simulink model "bicycle_sim"  (Simulink 10.2)
settings: Solver=VariableStepAuto  StartTime=0.0  StopTime=30  RelTol=1e-3
values from neighbouring files (symbols this model uses):
  a = 4    [bicycle.m]    (also in matlab.mat)
  d = 0.01    [bicycle.m]    (also in matlab.mat)
  Kp = 0.4    [bicycle.m]    (also in matlab.mat)
  Kth = 1.1    [bicycle.m]    (also in matlab.mat)
  Kx = 15    [bicycle.m]    (also in matlab.mat)
  Ky = 15    [bicycle.m]    (also in matlab.mat)
  L = 0.5    [bicycle.m]    (also in matlab.mat)
  theta0 = pi/2    (= 1.57079632679)    [bicycle.m]    (also in matlab.mat)
  w = 0.1    [bicycle.m]    (also in matlab.mat)
  x0 = a    (= 4)    [bicycle.m]    (also in matlab.mat)
  y0 = 0    [bicycle.m]    (also in matlab.mat)
libraries: simulink_extras x2
settings Model: Creator=olivier  LastModifiedBy=yukisaito
settings SolverCC: ZeroCrossAlgorithm=Adaptive
settings DataIOCC: SaveFormat=Dataset  SignalLoggingSaveFormat=Dataset
settings OptimizationCC: LifeSpan=auto
settings DebuggingCC: UnderspecifiedInitializationDetection=Simplified  MergeDetectMultiDrivingBlocksExec=error  MaskedZcDiagnostic=none  FcnCallInpInsideContextMsg=error  SFUnexpectedBacktrackingDiag=error  SFNoUnconditionalDefaultTransitionDiag=error  SFExecutionAtInitializationDiag=warning
settings HardwareCC: ProdBitPerPointer=64  ProdBitPerSizeT=64  ProdBitPerPtrDiffT=64  ProdLargestAtomicFloat=Float  ProdIntDivRoundTo=Zero  ProdEndianess=LittleEndian  ProdWordSize=64  ProdHWDeviceType=Intel->x86-64 (Windows64)
settings ModelReferenceCC: PropagateSignalLabelsOutOfModel=on
settings SFSimCC: SimUseLocalCustomCode=on
settings RTWCC: RTWUseLocalCustomCode=on
settings CodeAppCC: StateflowObjectComments=off
settings GRTTargetCC: TargetLangStandard=C99 (ISO)  CombineOutputUpdateFcns=on  GRTInterface=off
settings ConfigComp: CovMetricSettings=dwe  CovSaveCumulativeToWorkspaceVar=off  CovSaveSingleToWorkspaceVar=off  CovExternalEMLEnable=on

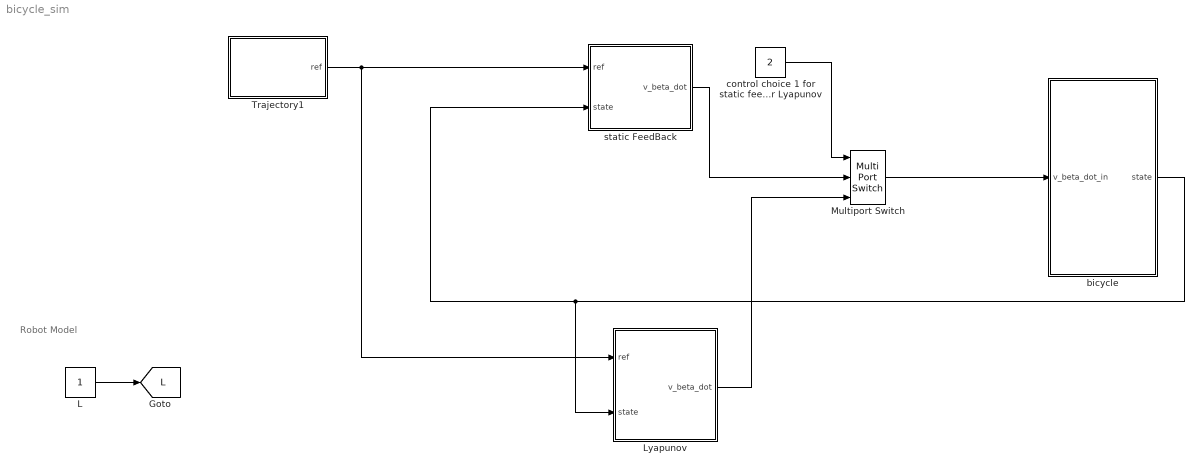
== system bicycle_sim ==
  note: Robot Model
  L : Constant
  Lyapunov : Subsystem
  Multiport Switch : MultiPortSwitch  Inputs=2
  Trajectory1 : Subsystem  TreatAsAtomicUnit=on
  bicycle : Subsystem  mask{L_error=0, radius_error=0, omega_max=100, beta_max=45, beta_dot_max=50}
      mask prompts: L_error "L error in percent"; radius_error "Radius error in percent"; omega_max "Max Rotation Velocity"; beta_max "Max Orientation"; beta_dot_max "Max Orientation Velocity"
  control choice 1 for static feedback 2 for Lyapunov : Constant  Value=2
  static FeedBack : Subsystem
  tag scope: L=global
  wires:
  Lyapunov/1(v_beta_dot) -> Multiport Switch/3
  static FeedBack/1(v_beta_dot) -> Multiport Switch/2
  L/1 -> [L]
  Trajectory1/1(ref) -> Lyapunov/1(ref), static FeedBack/1(ref)
  bicycle/1(state) -> Lyapunov/2(state), static FeedBack/2(state)
  control choice 1 for static feedback 2 for Lyapunov/1 -> Multiport Switch/1
  Multiport Switch/1 -> bicycle/1(v_beta_dot_in)

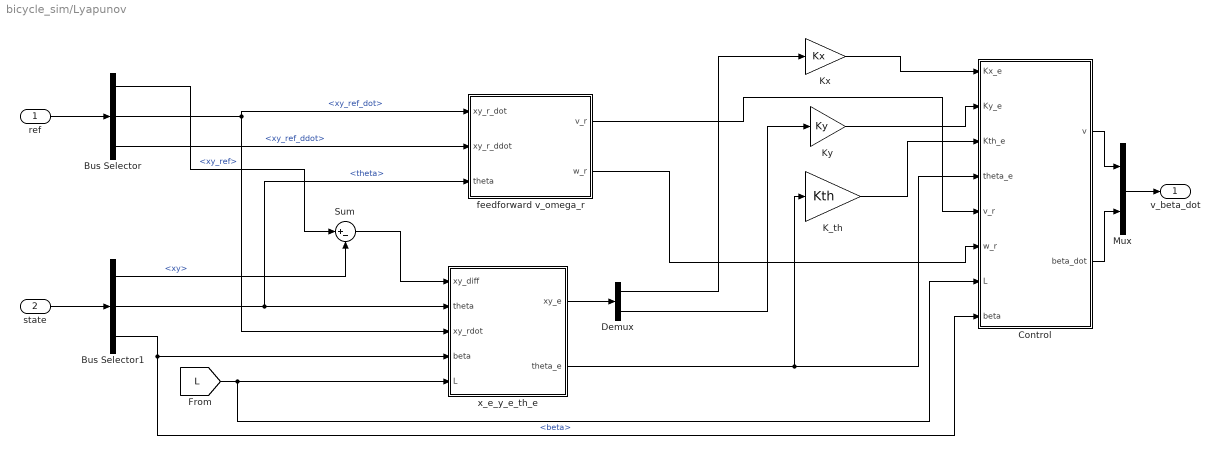
== system bicycle_sim/Lyapunov ==
  ref : Inport
  state : Inport  Port=2
  Bus Selector : BusSelector  OutputSignals=xy_ref,xy_ref_dot,xy_ref_ddot
  Bus Selector1 : BusSelector  OutputSignals=xy,theta,beta
  Control : MATLAB Function  TreatAsAtomicUnit=on
  Demux : Demux  Outputs=2
  K_th : Gain  Gain=Kth
  Kx : Gain  Gain=Kx
  Ky : Gain  Gain=Ky
  Mux : Mux  Inputs=2
  Sum : Sum  Inputs=|+-
  feedforward v_omega_r : MATLAB Function  TreatAsAtomicUnit=on
  x_e_y_e_th_e : MATLAB Function  TreatAsAtomicUnit=on
  v_beta_dot : Outport
  wires:
  state/1 -> Bus Selector1/1
  Demux/1 -> Kx/1
  Bus Selector/2 -> x_e_y_e_th_e/3(xy_rdot), feedforward v_omega_r/1(xy_r_dot)  "<xy_ref_dot>"
  Ky/1 -> Control/2(Ky_e)
  ref/1 -> Bus Selector/1
  Bus Selector/1 -> Sum/1  "<xy_ref>"
  Mux/1 -> v_beta_dot/1
  K_th/1 -> Control/3(Kth_e)
  [L] -> Control/7(L), x_e_y_e_th_e/5(L)
  Demux/2 -> Ky/1
  feedforward v_omega_r/2(w_r) -> Control/6(w_r)
  Sum/1 -> x_e_y_e_th_e/1(xy_diff)
  x_e_y_e_th_e/2(theta_e) -> Control/4(theta_e), K_th/1
  Kx/1 -> Control/1(Kx_e)
  Bus Selector1/1 -> Sum/2  "<xy>"
  Control/1(v) -> Mux/1
  Bus Selector1/2 -> feedforward v_omega_r/3(theta), x_e_y_e_th_e/2(theta)  "<theta>"
  x_e_y_e_th_e/1(xy_e) -> Demux/1
  feedforward v_omega_r/1(v_r) -> Control/5(v_r)
  Bus Selector1/3 -> Control/8(beta), x_e_y_e_th_e/4(beta)  "<beta>"
  Bus Selector/3 -> feedforward v_omega_r/2(xy_r_ddot)  "<xy_ref_ddot>"
  Control/2(beta_dot) -> Mux/2

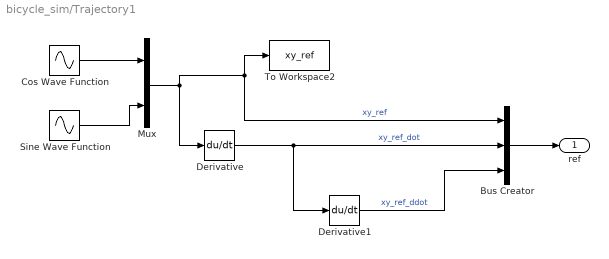
== system bicycle_sim/Trajectory1 ==
  Bus Creator : BusCreator  Inputs=3
  Cos Wave Function : Sin  Amplitude=a  Frequency=w  Phase=pi/2  SampleTime=0
  Derivative : Derivative
  Derivative1 : Derivative
  Mux : Mux  Inputs=2
  Sine Wave Function : Sin  Amplitude=a  Frequency=w  SampleTime=0
  To Workspace2 : ToWorkspace  VariableName=xy_ref  SampleTime=-1
      settings: Save2DSignal=2-D array (concatenate along first dimension)
  ref : Outport  VectorParamsAs1DForOutWhenUnconnected=off
  wires:
  Bus Creator/1 -> ref/1
  Mux/1 -> Derivative/1, Bus Creator/1, To Workspace2/1  "xy_ref"
  Derivative/1 -> Bus Creator/2, Derivative1/1  "xy_ref_dot"
  Derivative1/1 -> Bus Creator/3  "xy_ref_ddot"
  Sine Wave Function/1 -> Mux/2
  Cos Wave Function/1 -> Mux/1

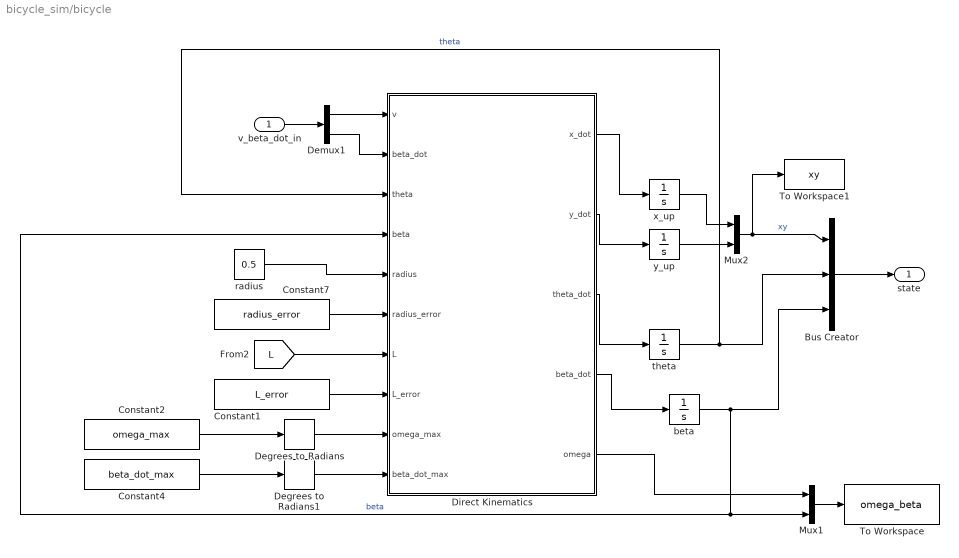
== system bicycle_sim/bicycle ==
  v_beta_dot_in : Inport
  Bus Creator : BusCreator  Inputs=3
  Constant1 : Constant  Value=L_error
  Constant2 : Constant  Value=omega_max
  Constant4 : Constant  Value=beta_dot_max
  Constant7 : Constant  Value=radius_error
  Degrees to Radians : simulink_extras/Transformations/Degrees to Radians
  Degrees to Radians1 : simulink_extras/Transformations/Degrees to Radians
  Demux1 : Demux  Outputs=2
  Direct Kinematics : MATLAB Function  TreatAsAtomicUnit=on
  Mux1 : Mux  Inputs=2
  Mux2 : Mux  Inputs=2
  To Workspace : ToWorkspace  VariableName=omega_beta  SampleTime=-1
      settings: Save2DSignal=2-D array (concatenate along first dimension)
  To Workspace1 : ToWorkspace  VariableName=xy  SampleTime=-1
      settings: Save2DSignal=2-D array (concatenate along first dimension)
  beta : Integrator  LimitOutput=on  UpperSaturationLimit=beta_max*pi/180  LowerSaturationLimit=-beta_max*pi/180
  radius : Constant  Value=0.5
  theta : Integrator  InitialCondition=theta0
  x_up : Integrator  InitialCondition=x0
  y_up : Integrator  InitialCondition=y0
  state : Outport  VectorParamsAs1DForOutWhenUnconnected=off
  wires:
  Direct Kinematics/2(y_dot) -> y_up/1
  Direct Kinematics/1(x_dot) -> x_up/1
  x_up/1 -> Mux2/1
  y_up/1 -> Mux2/2
  Mux2/1 -> Bus Creator/1, To Workspace1/1  "xy"
  Bus Creator/1 -> state/1
  v_beta_dot_in/1 -> Demux1/1
  Demux1/1 -> Direct Kinematics/1(v)
  [L] -> Direct Kinematics/7(L)
  Constant1/1 -> Direct Kinematics/8(L_error)
  Constant7/1 -> Direct Kinematics/6(radius_error)
  Direct Kinematics/3(theta_dot) -> theta/1
  Direct Kinematics/4(beta_dot) -> beta/1
  theta/1 -> Direct Kinematics/3(theta), Bus Creator/2  "theta"
  beta/1 -> Direct Kinematics/4(beta), Mux1/2, Bus Creator/3  "beta"
  Constant2/1 -> Degrees to Radians/1
  Constant4/1 -> Degrees to Radians1/1
  Direct Kinematics/5(omega) -> Mux1/1
  Mux1/1 -> To Workspace/1
  radius/1 -> Direct Kinematics/5(radius)
  Demux1/2 -> Direct Kinematics/2("beta_dot ")
  Degrees to Radians/1 -> Direct Kinematics/9(omega_max)
  Degrees to Radians1/1 -> Direct Kinematics/10(beta_dot_max)

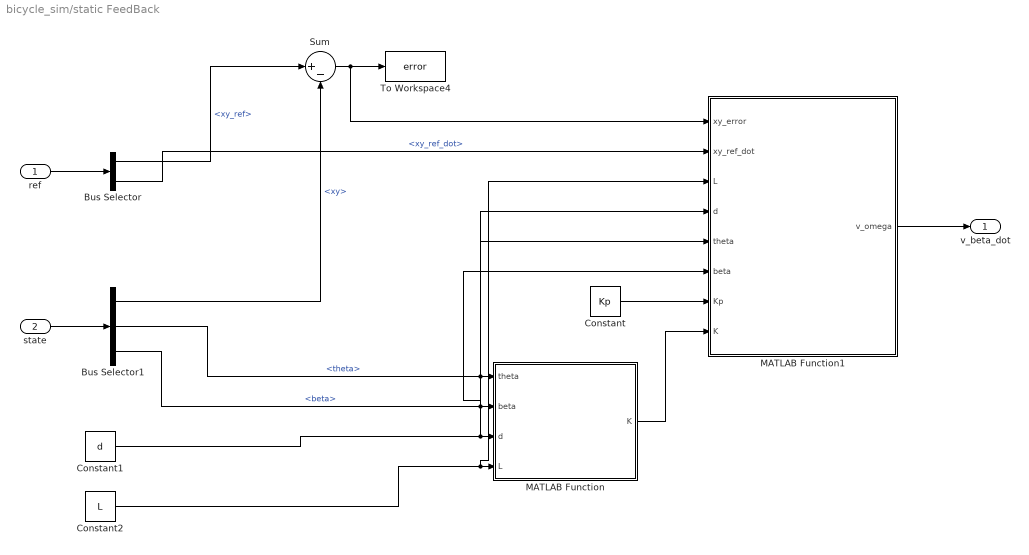
== system bicycle_sim/static FeedBack ==
  ref : Inport
  state : Inport  Port=2
  Bus Selector : BusSelector  OutputSignals=xy_ref,xy_ref_dot
  Bus Selector1 : BusSelector  OutputSignals=xy,theta,beta
  Constant : Constant  Value=Kp
  Constant1 : Constant  Value=d
  Constant2 : Constant  Value=L
  MATLAB Function : MATLAB Function  TreatAsAtomicUnit=on
  MATLAB Function1 : MATLAB Function  TreatAsAtomicUnit=on
  Sum : Sum  Inputs=|+-
  To Workspace4 : ToWorkspace  VariableName=error  SampleTime=-1
      settings: Save2DSignal=2-D array (concatenate along first dimension)
  v_beta_dot : Outport  VectorParamsAs1DForOutWhenUnconnected=off
  wires:
  Sum/1 -> MATLAB Function1/1(xy_error), To Workspace4/1
  ref/1 -> Bus Selector/1
  state/1 -> Bus Selector1/1
  Bus Selector/1 -> Sum/1  "<xy_ref>"
  Bus Selector1/3 -> MATLAB Function1/6(beta), MATLAB Function/2(beta)  "<beta>"
  Bus Selector1/2 -> MATLAB Function1/5(theta), MATLAB Function/1(theta)  "<theta>"
  Bus Selector1/1 -> Sum/2  "<xy>"
  Bus Selector/2 -> MATLAB Function1/2(xy_ref_dot)  "<xy_ref_dot>"
  Constant1/1 -> MATLAB Function1/4(d), MATLAB Function/3(d)
  Constant2/1 -> MATLAB Function1/3(L), MATLAB Function/4(L)
  MATLAB Function/1(K) -> MATLAB Function1/8(K)
  MATLAB Function1/1(v_omega) -> v_beta_dot/1
  Constant/1 -> MATLAB Function1/7(Kp)

== matlab function bicycle/Direct Kinematics ==
  data: v input double; beta_dot input double; x_dot output double; theta input double; beta input double; radius input double; radius_error input double; L input double; L_error input double; omega_max input double; beta_dot_max input double; y_dot output double; theta_dot output double; beta_dot output double; omega output double
function [x_dot, y_dot, theta_dot, beta_dot, omega]  = dk(v, beta_dot, theta, beta, radius, radius_error, L, L_error, omega_max, beta_dot_max)

% commanded wheel rotation velocity
omega = v/radius;
omega = max(-omega_max, min(omega, omega_max));

% actual linear velocity
v = (1+radius_error*0.01)*radius * omega;

% actual L value
L = (1+L_error*0.01)*L;

x_dot = v*cos(theta)*cos(beta);
y_dot = v*sin(theta)*cos(beta);
theta_dot = v*sin(beta)/L;
beta_dot = max(-beta_dot_max, min(beta_dot, beta_dot_max));

== matlab function static FeedBack/MATLAB Function ==
  data: theta input double; K output double; beta input double; d input double; L input double
function K = fcn(theta,beta,d,L)

K= [cos(theta)*cos(beta)-sin(theta)*sin(beta)-(d/L)*sin(beta)*sin(theta+beta) -d*sin(theta+beta); 
    sin(theta)*cos(beta)+cos(theta)*sin(beta)+(d/L)*sin(beta)*cos(theta+beta)  d*cos(theta+beta)];

== matlab function static FeedBack/MATLAB Function1 ==
  data: xy_error input double; v_omega output double; xy_ref_dot input double; L input double; d input double; theta input double; beta input double; Kp input double; K input double
function v_omega = fcn(xy_error, xy_ref_dot, L, d, theta, beta, Kp, K)

xp_yp_bias = [L*cos(theta)+d*cos(theta+beta); L*sin(theta)+d*sin(theta+beta)];
Kp_xr_xp = Kp*(xy_error - xp_yp_bias);

v_omega = inv(K)*(xy_ref_dot + Kp_xr_xp);

== matlab function Lyapunov/x_e_y_e_th_e ==
  data: xy_diff input double; xy_e output double; theta input double; xy_rdot input double; beta input double; theta_e output double; L input double
function [xy_e,theta_e]  = fcn(xy_diff,theta,xy_rdot,beta,L)
%#codegen

xe = cos(theta)*(xy_diff(1)-L*cos(theta)) + sin(theta)*(xy_diff(end)-L*sin(theta));
ye = -sin(theta)*(xy_diff(1)-L*cos(theta)) + cos(theta)*(xy_diff(end)-L*sin(theta));
theta_e = atan2(xy_rdot(end),xy_rdot(1)) - theta -beta;
xy_e = [xe;ye];
theta_e = theta_e - 2*pi*floor( (theta_e + pi)/(2*pi));

== matlab function Lyapunov/feedforward v_omega_r ==
  data: xy_r_dot input double; xy_r_ddot input double; v_r output double; theta input double; w_r output double
function [v_r,w_r]= fcn(xy_r_dot,xy_r_ddot,theta)
%#codegen

v_r = xy_r_dot(1)*cos(theta) + xy_r_dot(end)*sin(theta);

if(v_r ~= 0)
    w_r = ( xy_r_dot(1)*xy_r_ddot(2) - xy_r_ddot(1)*xy_r_dot(2) ) / (v_r*v_r);
else
    w_r = 0;
end

== matlab function Lyapunov/Control ==
  data: Kx_e input double; Ky_e input double; Kth_e input double; theta_e input double; v_r input double; w_r input double; v output double; beta_dot output double; L input double; beta input double
function [v,beta_dot] = fcn(Kx_e,Ky_e,Kth_e,theta_e,v_r,w_r,L,beta)
%#codegen
v = v_r * cos(theta_e) + Kx_e;
omega = w_r + Ky_e*v_r*sin(theta_e)/theta_e + Kth_e;
beta_dot = omega - (v/L)*sin(beta);
